simulink model "wrapper"  (R2024b)
settings: Solver=VariableStepAuto  StartTime=0.0  StopTime=100  RelTol=1e-3
settings Model: DataDictionary=wrapper.sldd  EnableAccessToBaseWorkspace=off  Creator=maciej  LastModifiedBy=maciej

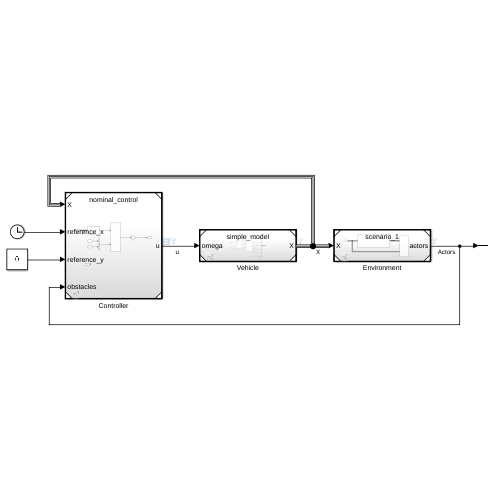
[thumbnail: Simulink's stored preview of the top-level diagram]
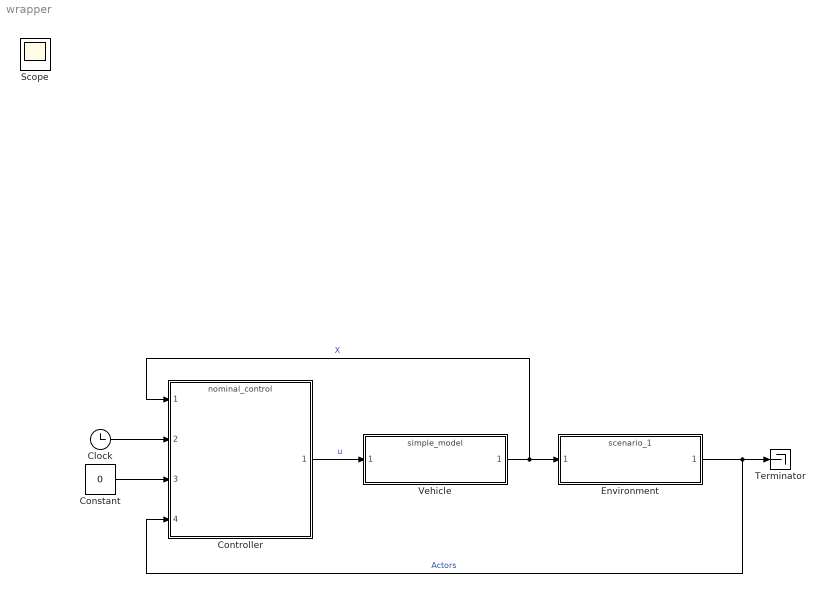
== system wrapper ==
  Clock : Clock
  Constant : Constant  Value=0
  Controller : ModelReference  ModelNameDialog=nominal_control.slx  SimulationMode=Normal  ModelReferenceVersion=1.48
  Environment : ModelReference  ModelNameDialog=scenario_1.slx  SimulationMode=Normal  ModelReferenceVersion=1.31
  Terminator : Terminator
  Vehicle : ModelReference  ModelNameDialog=simple_model.slx  SimulationMode=Normal  ModelReferenceVersion=1.17
  Scope : Scope
  wires:
  Vehicle/1 -> Controller/1, Environment/1  "X"
  Controller/1 -> Vehicle/1  "u"
  Environment/1 -> Controller/4, Terminator/1  "Actors"
  Constant/1 -> Controller/3
  Clock/1 -> Controller/2
